simulink model "CodeGeneration"  (R2020b)
settings: Solver=FixedStepDiscrete  StartTime=0.0  StopTime=inf  FixedStep=0.001  RelTol=1e-3  EnableMultiTasking=on
undefined symbols (not defined in the file or in its folder): batch3
libraries: TIMERS_Lib x7, neural x5, USART_Lib x5, STM32_Config_Lib x2, ADC_Lib x1, simulink x1
(part 1 of 2)
settings Model: SILPILModeSetting=veronly  CodeVerificationMode=processor-in-the-loop (pil)  ExtModeTrigDuration=10  Creator=anton  LastModifiedBy=anton
settings OptimizationCC: DefaultParameterBehavior=Inlined  EnhancedBackFolding=on  PassReuseOutputArgsAs=Individual arguments  ZeroExternalMemoryAtStartup=off  ZeroInternalMemoryAtStartup=off  MaxStackSize=64  OptimizeBlockOrder=speed  DifferentSizesBufferReuse=on  OptimizationCustomize=off  EfficientTunableParamExpr=on
settings DebuggingCC: ParameterTunabilityLossMsg=error
settings HardwareCC: ProdBitPerPointer=32  ProdBitPerSizeT=32  ProdBitPerPtrDiffT=32  ProdLargestAtomicInteger=Long  ProdWordSize=32  ProdHWDeviceType=STM32CortexM
settings SFSimCC: MATLABDynamicMemAlloc=off
settings RTWCC: Description=stm32 (Embedded Target)  SystemTargetFile=stm32.tlc  TemplateMakefile=stm32.tmf  GenerateReport=on  RTWVerbose=off  Toolchain=GNU Tools for ARM Embedded Processors
settings CodeAppCC: ForceParamTrailComments=on  IgnoreCustomStorageClasses=off  MaxIdLength=64  OperatorAnnotations=on  SimulinkDataObjDesc=on  SFDataObjDesc=on  CustomSymbolStrType=$N$R$M  SimulinkBlockComments=off
settings STFCustomTargetCC: CodeReplacementLibrary=ARM CMSIS SIN COS  MultiwordLength=256  ParMdlRefBuildCompliant=on  ConcurrentExecutionCompliant=off  IncludeMdlTerminateFcn=off  CombineOutputUpdateFcns=on  ERTCustomFileBanners=on  SupportContinuousTime=off  SupportNonInlinedSFcns=off  RemoveResetFunc=on  MATLABClassNameForMDSCustomization=Simulink.SoftwareTarget.ERTCustomization  CPPClassGenCompliant=off  GRTInterface=off  SystemTargetFile=stm32.tlc
settings ERTTargetCC: CodeReplacementLibrary=ARM CMSIS SIN COS  CompOptLevelCompliant=off  ConcurrentExecutionCompliant=off  IncludeMdlTerminateFcn=off  ModelStepFunctionPrototypeControlCompliant=off  CPPClassGenCompliant=off  UseToolchainInfoCompliant=off  ExtModeStaticAllocSize=256  ExtModeMexFile=ext_serial_win32_comm  ExtModeMexArgs=0,1,115200,10  InlinedParameterPlacement=NonHierarchical  ERTSrcFileBannerTemplate=sourceFileTemplate.cgt  ERTHdrFileBannerTemplate=sourceFileTemplate.cgt  ERTDataSrcFileTemplate=sourceFileTemplate.cgt  ERTDataHdrFileTemplate=sourceFileTemplate.cgt  ERTCustomFileTemplate=customRoutineProcess.tlc

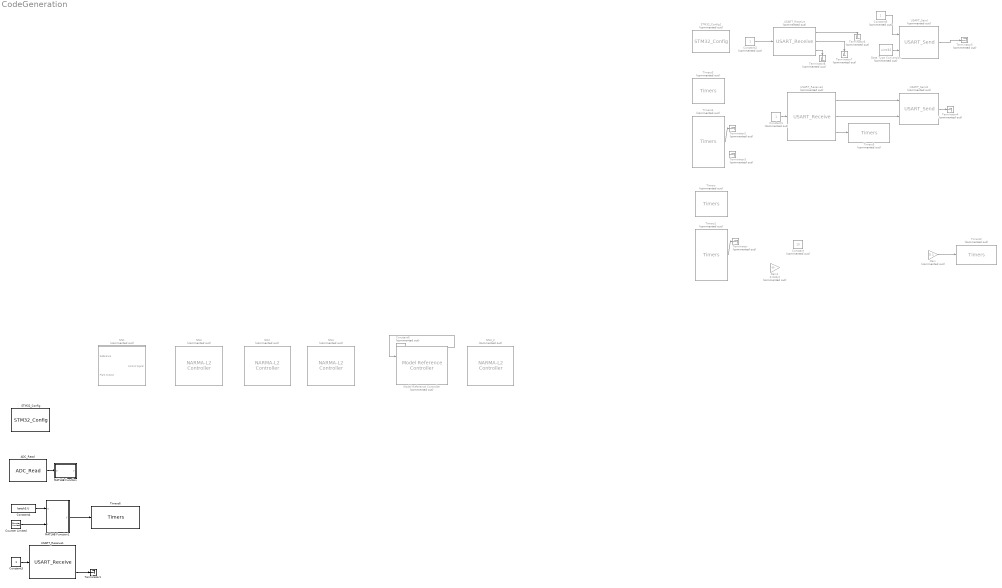
== system CodeGeneration ==
  ADC_Read : ADC_Lib/ADC_Read  ADC_Name=ADC1  ADC_Ch0=on  ADC_Ch1=off  ADC_Ch2=off  ADC_Ch3=off  ADC_Ch4=off  ADC_Ch5=off  ADC_Ch6=off  ADC_Ch7=off  ADC_Ch8=off  ADC_Ch9=off  ADC_Ch10=off  ADC_Ch11=off  ADC_Ch12=off  ADC_Ch13=off  ADC_Ch14=off  ADC_Ch15=off  ADC_Ch16=off  ADC_Ch17=off  ADC_Ch18=off  RgRk1=on  RgRk2=off  RgRk3=off  RgRk4=off  RgRk1_Ch=Ch0_r1  RgRk2_Ch=off  RgRk3_Ch=off  RgRk4_Ch=off  RgRk5=off  RgRk6=off  RgRk7=off  RgRk8=off  RgRk5_Ch=off  RgRk6_Ch=off  RgRk7_Ch=off  RgRk8_Ch=off  RgRk9=off  RgRk10=off  RgRk11=off  RgRk12=off  RgRk9_Ch=off  RgRk10_Ch=off  RgRk11_Ch=off  RgRk12_Ch=off  RgRk13=off  RgRk14=off  RgRk15=off  RgRk16=off  RgRk13_Ch=off  RgRk14_Ch=off  RgRk15_Ch=off  RgRk16_Ch=off  InjRk1=off  InjRk2=off  InjRk3=off  InjRk4=off  InjRk1_Ch=off  InjRk2_Ch=off  InjRk3_Ch=off  InjRk4_Ch=off  ADC_Trig=Not used  ADC_TrigEdge=Not used  DmaReq=off  DMA_Buffer=0  ItReq=off  AWD_Mode=NOT_USED  AWD_Ch=0  AWD_HThres=0  AWD_LThres=0  AWD_En_Int=off  AWD2_HThres=0  AWD2_LThres=0  AWD2_En_Int=off  AWD3_HThres=0  AWD3_LThres=0  AWD3_En_Int=off  EOC_SEQ=on  EOC_IT=off  JEOC_IT=off  AWD_IT=off  OVR_IT=off  CpltTrans=off  HalfTrans=off  ADC_RegNb=1  ADC_RegCh0=on  ADC_RegCh1=off  ADC_RegCh2=off  ADC_RegCh3=off  ADC_RegCh4=off  ADC_RegCh5=off  ADC_RegCh6=off  ADC_RegCh7=off  ADC_RegCh8=off  ADC_RegCh9=off  ADC_RegCh10=off  ADC_RegCh11=off  ADC_RegCh12=off  ADC_RegCh13=off  ADC_RegCh14=off  ADC_RegCh15=off  ADC_RegCh16=off  ADC_RegCh17=off  ADC_RegCh18=off  ADC_InjNb=0  ADC_InjCh0=off  ADC_InjCh1=off  ADC_InjCh2=off  ADC_InjCh3=off  ADC_InjCh4=off  ADC_InjCh5=off  ADC_InjCh6=off  ADC_InjCh7=off  ADC_InjCh8=off  ADC_InjCh9=off  ADC_InjCh10=off  ADC_InjCh11=off  ADC_InjCh12=off  ADC_InjCh13=off  ADC_InjCh14=off  ADC_InjCh15=off  ADC_InjCh16=off  ADC_InjCh17=off  ADC_InjCh18=off  NbADC=1  CurrentADC=ADC1
      settings: SourceProductName=Target Support Package - STM32 Adapter
  Constant : Constant  Commented=on  Value=10
  Constant1 : Constant  Commented=on  OutDataTypeStr=uint32
  Constant2 : Constant  Commented=on
  Constant3 : Constant  OutDataTypeStr=uint32
  Constant4 : Constant  Value=batch3.U  OutDataTypeStr=double
  Constant5 : Constant  Commented=on  OutDataTypeStr=uint32
  Constant6 : Constant  Commented=on  Value=20
  Counter Limited : simulink/Sources/Counter Limited  uplimit=15000  tsamp=0.001
  Data Type Conversion : DataTypeConversion  Commented=on  OutDataTypeStr=uint32
  Gain : Gain  Commented=on  Gain=0.1
  Gain1 : Gain  Commented=on  Gain=0.034/2
  MATLAB Function : MATLAB Function  TreatAsAtomicUnit=on  SystemSampleTime=0.001
  MATLAB Function1 : MATLAB Function  TreatAsAtomicUnit=on  SystemSampleTime=0.001
  Model Reference Controller : neural/Control Systems/Model Reference Controller  Commented=on  Nrc=[]  Nic=[]  Njc=[]  IW_y=[]  IW_u=[]  IW_r=[]  B1_c=[]  B2_c=[]  LW_c=[]  retraining_c=[]  max_i_int=0  min_i_int=0  max_r_int=[]  min_r_int=[]  Ts=0.2  S1=3  Ni=2  Nj=2  sim_file=0  trainfun=trainlm  Use_validation=1  Use_Testing=0  Use_Inc_training=[]  Use_previous_weights=1  max_i=100  min_i=0  max_r=[]  min_r=[]  sam_training=0  sam_training_c=[]  epochs=200  epochs_c=[]  minp=0  maxp=93  mint=21.399999999999998579  maxt=93  Normalize=0  IW=[-0.31575733105871184314 0.062686591686636455867;-2.3955199157333382858e-05 4.6988188726926723637e-05;0.64265348590034165888 -1.419013200965908883]  LW1_2=[-0.11494478982654444954 -0.21827174218633038638;-0.012095036588430245483 -0.011029687544739159855;1.3079273800536159733 1.1891128858228197096]  LW2_1=[-14.56571197986671784 -43.386573956542719088 0.012288416469105587631]  B1=[-7.6761807201422520563;0.70764088158851679022;0.8818915743236076521]  B2=16.065125218277426455  S1c=[]  Limit_output=0  min_output=0  max_output=0  Ref_file=0
      settings: SourceProductBaseCode=NN
  NN1 : Subsystem  Commented=on  AncestorBlock=neural/Control Systems/NARMA-L2 Controller  mask(NARMA-L2 Controller){Normalize=0, IW1_1=[0.081001796331336056722 0.15736369236145394956 -0.0061189171765253010798 0.031259373269709643528 -0.29161810270363336395 0.038960711989141236233 0.21066716241391639231 0.33564336592970134276 -0.42429187654869637836 -0.10771109383123129988 0.30271654934038322304 0.25669185229126045833 -0.18814574524270602507 -0.70360581796463639304 0.0022722054824509882454 0.22910624679545782412 0.31712007292734828434 -0.089593213208105274004 -0.29265065772660509014 0.25268525353674159417 0.40327134398474917543 0.10002475107419414591 0.10633957135057141297 0.22378520139222193852 -0.035441999466167897759 -0.09543965847989055451 -0.078475621102576539889 0.7978101624930962199 0.79197484966292575059 -0.75869567511731361709 -0.53133263705840783064 -0.40463183765462173991 1.4449740542986064806 1.423356606533091373 0.71567488745926521876 -0.71695273665588032941 -2.4976194364111630186 -0.52233538556271086328 -0.25784969469923535446 0.32001986891446365657 -0.34199391648141252986 0.21622613985873931353 0.51601933874237093658 -0.10229354784308368476 -0.063445068067935039835 0.76782685785385373922 0.58773337673444869811 -0.21322284745124506222 -1.3054574307789652554;-0.45565673055947875092 -2.8918895554005401571 -0.55732675097013917309 0.41047627061890573641 -1.0670853854999666765 -1.2269041735405823434 -0.53267398056508041826 -0.97207552132808006107 -1.5722657868604021925 -0.53941889635209872012 -0.032041342375024699229 0.09039551516666352593 -0.24629516613116916868 0.11927248975686825794 -1.2163427500639183432 0.94175325425605316276 -0.61664065600630824093 1.2537434811038190574 1.9708242434192153603 -0.18910074831646658811 1.1517160053052737378 -0.20615377037471419031 0.70037457310627138085 0.17251062422370158633 0.053382827490675487103 -1.651565422525036686 1.6906721755139886287 1.1022326413130534295 0.62515064205556036825 1.1201224089032946196 1.2824320188391788999 1.1251907270244796422 0.975294135970491749 1.2712381874161382544 1.8243027831043623355 -2.0127819149324448489 -1.9988806349665289019 0.0060280342477723233147 -0.028997473490317924455 4.2722776160136408663 0.96387017843053901522 -0.43562173505830670273 -1.0910256304234176028 -3.077903779867181111 -0.62300090522248086078 0.59335314064570743309 -0.10375978052824513798 -0.6895512783715659344 0.095697058256527731124;-0.042425975032530191533 -0.020290500259480211132 0.0020558665614247998224 -0.016851639980462271989 -9.5877759916884074858e-05 -0.00043919734009329294052 -0.02432381886257231618 -0.017583525777367700615 -0.017441386778719040335 -0.0040392297673593619001 -0.0038313554643087392899 0.0070579402620235629634 0.0078744850566811568082 -0.013939382367620677117 -0.0069330983391031903579 0.006428303090721439704 0.0076925694344603182118 -0.010213041618125990456 0.015297975743313978192 0.0069861958830649481533 -0.00039084881779854097235 -0.008621454336059724069 0.011403063240721680177 -0.027621446781558738753 0.0024782386744561469769 -0.0013077434278823262415 -0.00010498714836182009241 -0.0011898238650083332001 0.002668977180136910491 -0.00074960605879568792832 -0.0066212455474144917694 0.0036782537344367594902 0.0024779959822594154958 -0.0007716761197923681934 0.0060692515023587755713 -0.010470727481629332756 0.00651595757366603065 -0.0044179300248572807644 0.0023095130361779712264 0.0032279872975385253721 -0.0019027991455841971984 0.0030634915133303550032 -0.0039399868098482868778 -0.00029080766799168656462 0.0025879809946031118173 -0.00089996436815702825131 -0.0027431045461358116028 0.0015161575681175442926 0.00055000124936672957141;0.13973537349263717711 -0.030466654127967104926 0.13187207328935218742 0.08049426006455617788 -0.076243603851158442408 -0.16547014579527388745 -0.043008846385773881471 -0.11950007788257802077 -0.046614671001138807682 0.16047901716290213781 0.073120480998826051233 0.093856529495385407347 -0.24557469126930167591 -0.19531757450559239508 -0.25070881757410712343 -0.31477274386096759651 -0.23489476856896024382 -0.029056344281550659098 0.035279823771276613842 ...(+19340 chars)], IW3_2=[0.28221035721372655924 0.24949048164687237517 0.50091503695658035067 0.29138375416878581348 0.3047008394534790332 0.3601462353909597458 0.40525095161513946529 0.26607434365595128423 0.55636218982740370809 0.34241447621358733766 0.36922712946264368838 0.45012806085967455028 0.39746229989535664107 0.3517864672941124482 0.4414843841493564236 0.36597247241314873056 0.35722161160362497778 0.44166531166398254049 0.16265027540472642986 0.25024861114207264112 0.30989912765920363258 0.41245163179350691207 0.33932632574725996033 0.49564568667022140813 0.57942154725730332654 -0.41461285525358454462 -1.2532697594117170325 -1.016361035663570167 -0.50321252693688756086 -0.54111297537343439057 -0.64187004471658015703 -0.14877502282026722202 0.60233695514965923667 1.0051459831346829521 0.94121331461014512421 1.2528330966171683514 1.2616527525012983801 1.2522219802105709618 1.2306525532073226969 1.2285383897761898986 1.2223848740139509061 1.3599109870888566043 1.4151603107720585051 -0.24410711433607779064 -0.2618941587969862983 -0.29246174834972238354 -0.30083689664157564625 -0.3068812201344749413 -0.28850938424857819342;1.0039073009269712244 0.55909515429426293043 0.35983620274181782328 0.070909546265178188817 -0.31883710307836060638 0.021145812343666886557 -0.14052154577085901321 -0.3271388918228536058 -0.3056633047260269298 -0.1623172750176906376 0.27797165474081836356 0.15225869328795568758 0.07363456490444941771 -0.62576865843504525522 -0.049087382425018186161 -0.30920133067014099471 0.076637081473032608869 0.14304981128415980574 -0.036499429525520703244 -0.2347509035584434689 -0.26179516887628079269 0.31296574936306986725 -0.15475190365927896097 0.35308581539443995023 -0.10202609695406412993 -0.17396380085010321181 0.096710134721432985949 -0.20830070808662115578 -0.47058670424406728872 0.52295605161493230462 0.0094320573624777082067 0.06715455531127276223 0.04187265104715939823 0.30327034992914059242 0.20145747764813776159 2.0909735274704814856 0.84704439041569612456 0.50997408572182101327 0.30641972313442999987 0.19197087648156632711 -0.60791406184183405248 -0.59405380909595950634 -0.034990495138219557258 -0.069266505872329714455 0.21048086131964355294 0.22667210136932716691 0.042230258564031453172 0.03593561616959382865 0.053541505760580782036;-1.2112673056771381397 1.3552795429509238989 0.001340057277427330858 0.78347666775327995392 1.822361998970581709 0.5122989014137333541 -0.50111071047377020449 1.0617013213073929201 0.58128441457677981763 0.54344476225833260319 0.1944925038947179774 -0.43659907148292809165 1.707053424524483054 2.3777386093428747316 1.0594342712117987837 -0.35201497834900069561 -0.26906184398102572786 0.42788289669276663441 -1.4076861875310526795 0.19171855087256500783 -0.16925887294509342484 0.71966576151787531312 0.72059248245890283879 0.40053926618387347691 1.1464662234770182092 0.21463009737624402784 -0.80154327712810713447 -1.0629457174136294206 -1.0210941619912747846 -2.2004122602064311032 -1.9521985738729117354 -1.7172947022930669103 0.97621035059419447588 -0.44761702689860249915 0.77989707551171627564 0.40531267147789640237 1.1532982191938567773 1.1091066563735785255 1.4501837944712221429 1.6347891876696920566 1.3043885869211773176 1.4130197077664012895 0.91046411495307311146 -2.574445641552231212 -2.2214038450268880354 -2.6731230845813365171 -2.0029579616587414037 2.3026763340089528853 0.10442858352341162498;0.49547962694450214949 0.4634582007650282498 1.0890686566832370463 0.55177896616662225338 0.42636275537373924394 0.50771505829480712002 -0.12407657734639600255 0.32044081185938477763 0.81178540200128224136 0.43724654422399117371 -0.062071306632406897386 0.17905919149878501972 0.32630694572714147306 1.2520944876042674476 0.57891801858243330248 0.50502835376602539519 0.44893767424576869196 0.98344432483845856119 0.75591969357376931349 0.5511071553167703474 0.76629856245022498484 0.062215397882230967508 -0.15232706678745877582 -0.057308435995030514165 0.050820622281957550381 2.013762225413406437 ...(+18729 chars)], IW5_3=0.049794786120951804731, LW2_1=[0.019522040564175939525 0.010030780829141647259 -2.9269869808931687771 -0.044720248183330521541 3.3896735937268989147 0.055333660288906100222 -0.046769359291137894974 0.72657606414846986898 -0.231739559939226486 -2.8734140238129448619 -0.72738980090921023791 -3.1703753625289112783 0.030516532724820310402 -0.011164868475765466621 -2.6504898493220547806 -0.017243119800886514553 -3.6192209431664785768 0.062752740912268317741 -3.4737778709395779053 -0.020630211384971723632], LW4_3=[-0.49767595711144158033 -5.0418393908440179985 3.5744239145482166187 -3.9384524981309438907 -4.8073499402252970469 2.727310872235649164 -0.71730478292060606549 0.12740639700024902758 -4.6201956999409405924 4.0234022300950194051 5.8975918809235290396 1.9099313228049630276 0.22431709645351263771 4.1350604422295358376 3.8128713144263901569 5.2889865099553734495 5.1501748174827808313 -2.0783275816180553086 0.87022382331586878301 5.2226018567932683823], LW5_4=0.25213902069175248011, LW6_5=-0.0018683962758275409616, LW6_2=1.0196993926720294699, B1=[-13.683970472853349776;-10.829168374571350952;3.2499778850305398592;12.860073554387984274;-4.3007772967563742128;-12.715349009048415141;6.4787516301547949382;-19.564844579552055137;0.20783599937462277074;-5.7023611773114426526;10.113035508787838523;13.286447344365756251;2.8802714807787950235;26.296794390935232855;-0.69066711291984395071;-0.52575739785160779949;-8.8606049427338184898;-14.753008137324961524;1.7681866839940678648;10.252069531512537637], B2=3.7097017031416461563, B3=[0.15043469453056407259;2.9756978074974016479;7.1920582605238250196;-9.8267085343876328096;-1.1888977589751141828;-10.309826346565044375;-5.3298483838539478796;6.2524100723987032779;-3.1661464323339654214;-10.512300523957687659;-10.477978044887745313;-9.6945816023752779955;-15.116599806060138533;11.336838798593424471;11.996325424358646572;-0.47776234751081703145;6.2912996815758619462;2.9850645554334387377;2.5315214878778347085;19.896605647385079862], B4=2.3815464859015680332, Limit_output=0, min_output=0, max_output=0, Use_Previous_Weights=1, Ts=0.05, S1=20, Ni=25, Nj=25, sim_file=0, trainfun=trainlm, Use_validation=1, Use_Testing=1, max_i=100, min_i=0, max_i_int=0, min_i_int=0, sam_training=0, epochs=100, minp=4, maxp=94, mint=20.899999999999998579, maxt=94}
      mask prompts: Ts "Sample time"; trainfun "Training function"
      mask help: NARMA-L2 Controller. You first train a neural network model of the plant to be controlled. The controller is a rearrangement of the trained plant model. Double-click the NARMA-L2 Controller block to begin the plant training.
      mask init:
      | network;
      | x1 = [0    .4   NaN  .33  .55   .55  .33  .33  NaN .80  .92 .92];
      | y1 = [.95 .95 NaN  .75  .75   .55  .55  .75  NaN  .95 .95 .65];
      | x2 = [0    .43 NaN .45 .45    NaN .92 1.2 NaN .63 .85 .85 .63 .63 ];
      | y2 = [.39 .39 NaN  .41 .55   NaN .65 .65 NaN .75 .75  .55  .55  .75];
      | x3 = [.45 .45 NaN .42 .45 .48  NaN .33 .4 .33];
      | y3 = [.75 .90 NaN .83 .90 .83  NaN  .98 .95 .92];
      | x4 = [.75 .75 NaN .72 .75 .78  NaN  .5 .7 NaN .63 .7 .63];
      | y4 = [.75 .90 NaN .83 .90 .83  NaN .95 .95 NaN .98 .95 .92];
      | x5 = [.43 .43 .77 .77 .43 NaN .36 .43 .36 NaN .75 .75];
      | y5 = [.37 .41 .41 .37 .37 NaN .42 .39 .36 NaN .41 .55];
      | x6 = [.92 .92 .77 NaN .84 .77 .84];
      | y6 = [.65 .39 .39 NaN .42 .39 .36];
      | x1t=.03; y1t=.31;
      | x2t=.03; y2t=.85;
      | x8t=.03;y8t=.21;
      | x3t=.77; y3t=.53;
      | x4t=.77; y4t=.44;
      | x5t=.34; y5t=.49;
      | x6t=.58; y6t=.49;
      | 
      | 
      | t=(0:24)/24*2*pi;
      | xs = .05*cos(t);
      | ys = .05*sin(t);
      | xs1=xs+.45;
      | ys1=ys+.95;
      | xs2=xs+.75;
      | ys2=ys+.95;
      settings: OpenFcn=nncontrolutil('nnident','',gcbh,gcb,'narma_l2');
      mask Help: helpview('deeplearning','nnet_narma_l2_controller');
      mask TypeOptions trainfun: trainbfg | trainbr  | traincgb | traincgf | traincgp | traingd | traingdm | traingda | traingdx | trainlm  | trainoss | trainrp  | trainscg
      mask Display:
      | e = 0.06;
      | c1 = [120 150 230]/255;
      | c2 = ([120 150 230]+0)/383;
      | c3 = ([120 150 230]+128)/383;
      | patch([0 1 1 0],[0 0 1 1],c1);
      | patch([0 1 1 1-e 1-e 0+e],[0 0 1 1-e 0+e 0+e],c2);
      | patch([0 0 1 1-e 0+e 0+e],[0 1 1 1-e 1-e 0+e],c3);
      | plot([[x1 NaN x2]*.9-.075 ], [[y1  NaN y2]*.9-.1 ]);
      | plot([[x3 NaN xs1 NaN xs2]*.9-.075 ], [[y3 NaN ys1 NaN ys2]*.9-.1 ]);
      | plot([x4 NaN x5]*.9-.075,[y4 NaN y5]*.9-.1);
      | plot([x6 NaN ]*.9-.075,[y6 NaN ]*.9-.1);
      | plot([0 1 1 0 0],[0 0 1 1 0]);
      | text(x1t,y1t,'Plant');
      | text(x8t,y8t,'Output');
      | text(x2t,y2t,'Reference');
      | text(x3t,y3t,'Control');
      | text(x4t,y4t,'Signal');
      | text(x5t,y5t,'f');
      | text(x6t,y6t,'g');
  NN2 : neural/Control Systems/NARMA-L2 Controller  Commented=on  Normalize=0  IW1_1=[0.42999578451454106842 0.20519526356674350209 0.48560842768546641501 0.45796392885806858075 0.56450148087544238518 0.50351630398968461044 0.40693748816290253867 0.42403535086980548297 -0.58936365396049317233 -0.30903885679007220277 -0.22292526287955208297;0.25841032509566608244 -0.13737805067406735904 -0.15482151715535916181 0.65297703160385611731 0.17274411066130934689 0.40453996700577132817 -0.4111114686333410817 0.36147208605498298839 0.021131113938576966127 -0.14014771021062302769 0.092839271051875879581;-0.011434700121978670986 -0.010720729619677252242 -0.0096564374143097118919 -0.0082604891885513388045 -0.0096005768011547358565 -0.010391114612203487463 -1.0476759531353016286e-05 7.2077522336085755677e-05 -9.6420386119362220373e-05 8.2917824210678723652e-06 2.3416884195674133776e-05;-0.56744746474663465552 -0.47940353954936382186 -0.36673868830426242793 -0.72388284193056895433 -0.22890654036687180239 -0.62816667955451999106 -0.15556880492137584171 -0.27089640898497230337 -0.1535093393110727733 -0.72590483691104790154 -0.80082100631588459816;0.63814745459816246687 0.6401406546649579532 0.26654247833268734924 0.2952640512926372196 0.84955032500919014371 0.21317123129875506504 -0.29465041983107009838 -0.19037508756029189461 0.15397062431184516118 -0.07918764571200906377 -0.049066929249987248363;0.68031528203635949215 0.37921354169754795116 -0.022222469467425922524 2.0972653722608960436 0.40664857275118748703 1.4365602546419606877 0.16120398009003295003 0.033632347331193010453 -0.20163202670797347738 -0.58984661369907187556 -0.91883922634755954562]  IW3_2=[0.62072958787989240825 0.48642642668883517842 0.8143032356552284412 1.1295518407252980175 -0.12252819519746503685 1.3035863364893975902 -0.061540668235754963922 0.13396836381379054193 -0.97273489523940537271 -0.57449054628195250771 -0.79552860018882165516;0.022148742001209309471 0.35509226217601974618 0.15936552561537462025 0.41743348717457334773 0.21671159251167160242 0.21588238211386889809 0.10365014565444288785 0.32399157654972332576 -0.24370824872351357082 0.1052740296345326676 0.21533119379063728194;-0.34960873325137170609 0.60597565806765596452 1.122135647654741053 -0.20643521097916414653 0.71677006726172487472 0.30105254139888160125 -0.12032940047543728979 -0.37497085528307366742 0.34043889151749706645 -0.36823126955913926261 -0.11653268522074718139;0.19393773260013844051 0.067610881920749932306 0.23399090778869918728 0.21457707930399366747 -0.14374410046381749795 0.26692484357754975299 -0.17370341744012737784 -0.06060480970759270225 0.25309705955902561669 0.086487428730836077295 -0.042775161104023948222;0.97957315902225849946 1.1975315558082157974 0.94192073634989559316 1.2208743757048998724 1.3045447227043793781 1.0252258514225500718 0.17267256498501859507 -0.27917778045509750173 -0.21332665529313060704 -0.94663326100635658555 -1.4586763385411685157;-0.13919708229624574991 -0.04346517225565629805 -0.26370853710094882549 0.28690607977414084306 -0.38642813425088834434 -0.033589343275048713644 -0.02182821320742767135 0.0546643245090925739 -0.093743190688845248748 -0.083182309228358813913 -0.23796081789112336069]  IW5_3=0.00035625599399004379431  LW2_1=[0.0097832663468938908802 -1.6727188551373248782 4.0745823001807295327 0.70095287853249088617 -1.5696668938645457203 -0.0037480653401194630528]  LW4_3=[-1.3975705228945904945 0.5017185102204857472 2.1171483657331444661 -0.28696914872047785128 -0.97527522346300143941 0.42327247399147505114]  LW5_4=0.30108920563813407201  LW6_5=-0.64763974290970649506  LW6_2=-4.0888519730117227624  B1=[-12.820258601526894893;8.3658161662943157921;1.4697304281208545262;2.3120851336475483073;-3.5099662930913710923;-7.2883678124612831795]  B2=-2.0492682323172446424  B3=[-12.875713784252596383;-2.8354269756645469336;-6.0083619963053065405;-3.7653708851426892501;5.4665583507364479132;7.3625549242107526382]  B4=-0.58721073754749031348  Limit_output=0  min_output=0  max_output=0  Use_Previous_Weights=1  Ts=0.05  S1=6  Ni=6  Nj=6  sim_file=0  trainfun=trainlm  Use_validation=1  Use_Testing=1  max_i=100  min_i=15  max_i_int=0  min_i_int=0  sam_training=0  epochs=200  minp=18  maxp=98  mint=21.600000000000001421  maxt=98
      settings: SourceProductBaseCode=NN
  NN3 : neural/Control Systems/NARMA-L2 Controller  Commented=on  Normalize=0  IW1_1=[4.5877506179710243472 -5.8224880884168586093 -4.8116398201014956015 -1.4164815216642832052 0.81763038785532338171 -0.27198057915801182594 2.0143444159160965867 2.3407559126241523906 -1.7681452057802877764 -5.7821022484229143146 3.7430851758116423511 1.6721227367707509615 1.3289005909715654319 0.93538382702478350961 4.3919906169554563391 2.8708971599556645238 2.9337230728926533274 2.9439570630901070736 0.89485599525993375636 0.85017517791716412656 0.86891756124519170523 0.84581278816392069242 1.4448529792500321989 -2.2530121666458060581 -2.2394658222812600101 -2.2623666698858242441 -3.2386103949984401673 -2.8441633821784511049 -3.0600299960223735773;1.1720830805014157416 0.72510029776086915021 3.1152837564444717522 0.18904910378056175024 3.8224935256831891195 -1.9668126489800641377 -6.6675532679147675452 3.2650850036067073923 1.1202470114644642596 -6.2278464287587462778 3.7116215488970412117 -6.0685565334704545393 -5.0774544557597840466 -2.8632327825585677239 -0.26624337447103779697 2.8212503138002418268 -2.508547996937386948 -1.5743516070179877087 -1.3523844495695789281 -1.7764149308941030725 0.61474795424465311644 0.70076912677360470028 0.81227561839137796262 3.1740642999768993171 12.312848336435406438 12.355930113796736336 -7.2886823026066540621 -7.2809179605649720912 -7.2988342602487490396;3.0430016330075329023 2.4169740318724475259 2.4259277921412216728 4.5817733742367368066 1.8944438398997343054 1.859511580790785823 -0.53850317948302839355 -1.8306580945271937466 -1.2368319834834635706 -4.0322762699266911923 -0.2109757274893888368 1.9557147957371048275 -4.01940545609330524 -2.9868338460211498742 -2.6261247205624504986 -4.6830705275812238852 1.3397092110462973658 1.6504232012093991155 3.4069702118395546186 -3.22513040401769846 -3.4683445151905072379 -2.7658917471572559421 7.3974017903997095758 -1.5641115142871362398 3.7003543748091578536 -5.2653694153891770213 0.44047543295537849861 0.65058131350162340389 1.7225709767556538488;-4.890279222734382536 9.2820623635560259856 6.5998750720783911916 6.0323139426130865104 -5.0047680067878452803 0.4116948987745852051 -6.2914181154535384621 0.31808446778836885205 0.26438247585563112718 8.3922146620896498348 -4.7408709297709625829 2.9144904287601018922 -4.6124591317731447049 -6.1094582691993482015 -11.011217763455704244 0.27404268366330397644 0.55924390847268445892 0.46783190716662831354 0.70671702031784744413 0.73672189036226576331 0.61756628614558117807 0.78035668849300543481 0.78927769025750360576 0.81077837110447059654 0.81143931394686774627 0.74610299054055284618 0.97731444593670147025 1.0958561553222312401 0.90844578056274372102;-0.075236161728419265193 1.4529627010312577973 2.797812619081362584 3.5136868279571298324 2.7611251052148499951 2.4983963255208156973 -1.7656841404250225303 -1.9417134095882566669 -0.78088116642014793189 -1.6088640550687902664 1.7943691324232813322 0.94997145365046986587 -4.1264897357333518713 -0.026775423540358334051 -1.1477510773823724755 0.50378607124498253622 1.6560927415077055791 2.0531450920801437299 1.8745776862605858515 -2.0491210315044381396 -1.5608325026743929964 2.5284665887730941591 6.2502127026131972798 -10.694048550901566585 52.122961578317422493 53.556309256001412678 -36.106296288576920972 -36.030576479366580145 -36.593007834026053615;0.063989575652429978025 -0.041556986550670353686 -0.031083652266411285203 0.066651685652164505136 -0.041734549960076069985 -0.039025355723310617417 0.11953734079408176449 -0.085248904267280753433 -0.094181208689583476024 -0.033628899970372320982 -0.096945136753965252541 0.064131397883877019894 0.094625341370090709781 0.014827917287662261553 0.022585848901328225979 0.032759617241095002893 0.086220411041693659215 0.036976528993942395229 0.0092108912715153350853 0.06098449913498683872 0.034752769386083626202 -0.0051608948789154344278 0.0030326550159277270054 0.03485484675740441185 0.020253180352680037052 0.022824635982994119499 0.062310072838543721641 0.049798250842962854534 0.05015314426113818419 ...(+6138 chars)]  IW3_2=[0.062358389312379768066 0.059933867760648178169 0.059638039922337023058 0.039257799225629746998 -0.042892977608521710986 0.0087672609423849329202 -0.088440379294083742989 0.0043407700365922161079 -0.069881551551252293897 -0.088294496696273705449 0.041782477480814379789 0.059899181680647554937 -0.053645572449268187631 0.0028564156442049942058 0.078278081841138769104 -0.062008991991044801195 -0.053842263884374699789 -0.056195992817942741482 -0.034043222959654229065 -0.05050491174069139666 -0.038932059557208006928 -0.036324361972531811482 -0.019517496463399789525 -0.035456060620168178277 -0.012989875113196928946 -0.032487776126200282323 -0.001676689509518164943 -0.03667993303948401812 -0.029093856497292583385;0.0089341949146411227256 0.043196542765014042664 -0.046111763793666681044 -0.010471157526264679438 -0.062364231135924583227 -0.069121549529261222533 -0.060856269400886821297 -0.042418400517974581831 -0.060451262386795656667 -0.058346796047875681968 -0.079180222859112261991 0.0036802027370557398311 -0.043534445102530884564 0.0032102009835526211512 -0.017187221611705216784 0.15476161783268815864 0.12419758316213640181 0.1509952992578698916 0.14900803654666891496 0.13627369075906650697 0.11927773201766439515 0.14707599051007264057 0.13143743150228534566 0.13213462714122772845 0.13648149315145291505 0.13219979331239042897 0.1113272258290868566 0.14440329380429550721 0.142947377058244951;0.12046319339193144182 -0.052836313895128696194 -0.18981219103144658655 0.14408618432149167266 0.10276892132357731691 0.02656259847398110413 0.22292100843881473837 0.0057495277134840400146 -0.064435903389781640227 -0.0754980337842851984 -0.017866303955107208645 0.061765817288670116225 0.094341894661344016804 0.045483043120726859843 0.069462039727850921622 0.2331143029282263246 0.17268281646288186071 0.20025995022356612996 0.16257429492522024184 0.16567807576394280589 0.11476257681776874664 0.18090963329736181597 0.167073510298331257 0.14080977051149509705 0.12020884580905538686 0.14531005680825850868 0.021790618609190737232 0.11039150224340435469 0.11247882883628886053;-0.15739762904048695824 -0.25478239310084827007 -0.23853135867673710968 -0.24540693320706696845 -0.16549847789694849265 -0.27158208680699980064 -0.21228824520764491557 -0.19678463023799608322 -0.26334512571602797237 -0.26091440994101733342 -0.17703690068545505087 -0.16062972508328765553 -0.17598358115945855751 -0.1625496424016726893 -0.26635838210801798809 -0.208884459953958046 -0.1958764217202477731 -0.22208704458775718749 -0.20691536192094434066 -0.19469013205881979811 -0.18973203077934586158 -0.19296929867747744658 -0.20934125304262610201 -0.18182131675118293201 -0.57697276897127347528 -0.56119084851973710659 -0.5444357114933243702 -0.55980672953996235552 -0.54540635348844834773;0.24513278189851642197 0.20116485478010875942 0.25106234233440560821 0.16428185090259478374 0.27637620423829373228 0.30473283233506875955 0.28957088935705294075 0.31127710182372531067 0.18963656982560209152 0.28772079439633801989 0.30936472356509092663 0.27728849140228650771 0.29554353755051698815 0.25561277516872132898 0.21826262337416668657 0.2385315486962933107 0.23053664672280740899 0.23024892752520442762 0.20902791755162322684 0.23984961740448723644 0.22641550141436861399 0.23291025382129931787 0.20466253945367876566 0.16332858598416366558 0.22964847146070285766 0.23807019566036549674 0.2312341398611621468 0.20592225130579747128 0.22734686274357324143;0.10380903006185050741 -0.010075763651438730817 0.0052896867225735964835 -0.0069488036995434578069 0.073615356241652343816 0.11093664740531761215 0.1038982260322044715 0.03694189997265746872 0.047896550304743219784 0.12812174606833567903 0.13676691363433837734 0.022426014661011049039 -0.056927337711005866761 0.053972174985606441444 0.10425328952949819428 0.047670282041615913426 0.047302942221664076583 0.067193549163231794386 0.073391657383844760565 0.050650439670443012097 0.081544057044356729747 0.0792206487885007693 0.061724658743079800771 ...(+6400 chars)]  IW5_3=-0.40683118950996954855  LW2_1=[0.18367388632745329513 -0.24113376646743667209 -0.18732164710016388498 1.1048657870521041424 0.76391327859509616793 4.864930235214743881 0.59561883111477309516 -1.917303539599590323 -4.5862699562656992214 -1.1489886963737321324 0.50461435467110316022 0.48671555729633336762 0.78282586687516497737 0.17113935506526886665 -4.5042654176370335861]  LW4_3=[-0.24550482457143141257 -0.12046258227206883828 0.72278059400088856545 0.33556409988396906918 -0.20365096582041067319 -0.11065065970533820294 -0.39702006218300750495 -0.16909710388117193958 0.19457023564358214007 0.20368125579817983328 0.71902791528125675757 0.27180791243058466389 -0.62803781344313702739 1.0228245811182321567 0.24864886041124215077]  LW5_4=-0.704032194384420551  LW6_5=-0.00052115716235789574795  LW6_2=1.4812383354715947803  B1=[6.6037858506714020024;15.6190590967843832;7.2115002157788001824;4.6111630565620940203;-5.8133616172725615101;-0.61352439361774413484;-16.867912000695010732;11.523777125561503354;0.42855780624155320746;5.9314288248581084062;4.7460568926869948214;134.65286029529784173;-8.0407779755833939106;6.4517055479975411458;1.1610416736300694929]  B2=3.607603047460834933  B3=[-7.1527970321948846077;8.1273504245326648743;-6.6030087185907824221;1.1987536425192513168;-13.393850128780036002;0.62586972328921175457;1.2876737461148741737;-0.63156149919191872932;5.704177607140747952;-8.8977463766610807028;0.75364248725632110304;-11.922694834115555196;4.1889470813052707143;1.0906150890423740307;8.2092594533763563192]  B4=0.8861775603168042803  Limit_output=0  min_output=0  max_output=0  Use_Previous_Weights=1  Ts=0.05  S1=15  Ni=15  Nj=15  sim_file=0  trainfun=trainlm  Use_validation=1  Use_Testing=1  max_i=100  min_i=0  max_i_int=0  min_i_int=0  sam_training=0  epochs=200  minp=27  maxp=89  mint=20.399999999999998579  maxt=89
      settings: SourceProductBaseCode=NN
  NN3_2 : neural/Control Systems/NARMA-L2 Controller  Commented=on  Normalize=0  IW1_1=[0.039148714389914393563 0.04184575771883371903 -6.0296183153573701169e-05;-0.34244510037897918364 -0.83577023563736208001 -0.98984885365635955079]  IW3_2=[1.7482699976429136868 1.6815146793184658769 1.4643769373344286411;0.19971534547986175001 -0.23761110741996102624 -0.8313049704497363912]  IW5_3=0.0022432448317685066419  LW2_1=[2.4678568562519433982 -0.92133163820607499872]  LW4_3=[0.40163841185159132596 1.6230344928063593635]  LW5_4=-0.69253692308886294349  LW6_5=0.30756804882471866502  LW6_2=5.0314703685039310344  B1=[-2.061019820097664379;12.38881103090871072]  B2=4.1381115783143034292  B3=[11.273095141969324828;-4.8446886512396289959]  B4=0.11102912396311917509  Limit_output=0  min_output=0  max_output=0  Use_Previous_Weights=1  Ts=0.05  S1=2  Ni=2  Nj=2  sim_file=0  trainfun=trainlm  Use_validation=1  Use_Testing=1  max_i=100  min_i=0  max_i_int=0  min_i_int=0  sam_training=0  epochs=200  minp=27.030000000000001137  maxp=88.780000000000001137  mint=22.440000000000001279  maxt=88.780000000000001137
      settings: SourceProductBaseCode=NN
  NN4 : neural/Control Systems/NARMA-L2 Controller  Commented=on  Normalize=0  IW1_1=[-0.080988746250572979379 -0.13838781841168235065 -0.19464246714003791139 -0.1831737734679177998 -0.2549585151304777364 0.11295712996615900336 0.05396774551908024159 -0.084339983840538590432 -0.099785442419433004191;-0.010413890184333134126 -0.0091265575187428824022 -0.0063756329127272279994 -0.0083552108579549901057 -0.006076863504177858373 -9.7817671395440236029e-05 8.1153955099971645821e-05 9.715541730819373886e-05 1.7392127962488782369e-05;1.1513020654288714795 0.94415618342208462721 1.0375567840161767919 1.1229222945685994883 0.99225626847447712109 -0.1672127966254446374 -0.58243645017103307104 -0.43951626273631466679 -0.46180103710983733123;0.31910512731660528596 0.18870905461896675392 0.30841530355997776036 0.2982128793490136931 0.15411073386352708292 -0.029105687147781077184 -0.025462669894502486245 0.074244400452648851019 -0.17206703549074439663;0.28332045741420497365 0.25883705328865552753 0.55734588837675969053 0.45118178103568723492 1.1993033791487037742 -0.35307827846730166499 -0.046426401736290534572 -0.093962967387348550474 -0.34001905894463368973;0.63303424346071923701 0.61938341492344972661 0.67256845103291218457 0.69445647014096156813 0.75938987527353773999 0.47173708842661332685 0.485307212211659178 0.74210755204577560917 0.89534925039593660223]  IW3_2=[0.44433842822056818234 1.3308322142928747933 -0.88012309141376154908 0.10209499927550060028 -0.88668043204048252459 0.53298752161663853766 -0.016887785036579797127 -0.10699666035565690014 -0.43642222102782957105;-0.014213960576156930635 -0.98861648612602792685 0.62704188928941684278 0.19568832301796451612 0.13346564627213525212 0.1777508676739525395 0.10747435497132751259 0.34252847506430900149 -0.25680987507368963074;-0.15706502702782226821 0.18298497505928557061 0.035550919971730599034 -0.1396805708606352614 0.75028649860879381706 -0.0025150096985902493582 -0.088907366005240601181 -1.3441539181459039032 -1.3790216143720746;-0.23978469641887353858 -0.17759817661117477394 -0.17920698162589127067 -0.11455427433702475293 -0.0065057513890076018939 1.0272449657783668808 0.054508489687626650311 -0.032900514715066796201 -0.96858067035532324773;0.054410824928441445247 1.135534700071001657 -1.1676159002227570749 0.20397275271952425291 0.30242317544510588512 -0.027482815395496559829 -0.17393561909169577562 0.26424641101867157866 -0.074329744658186397421;0.08744818385947852879 0.095150012693570609756 0.059360282314576982843 -0.034850119895690243044 -0.057757247277703628596 0.2336660396468579759 0.19464318987828485574 0.15883347432507274877 -0.017678744283946268984]  IW5_3=-0.13699552970148068387  LW2_1=[1.1337981223783673013 5.2120259965505066901 0.029738112641827050414 -2.0044783267070078736 -0.034367633415846428335 -0.40681614747368238794]  LW4_3=[-2.1127949727651209599 -0.12122275336356981568 -0.91255569383502321834 0.010290064043029454807 0.66342205934284392832 0.60424499164512324167]  LW5_4=0.0076462523402957864246  LW6_5=-0.23311673795632711914  LW6_2=-4.7659452310226351202  B1=[5.5401485961125951363;1.114108857171022704;11.704355155680048028;-3.6962123711345546972;3.3365644845355144632;2.3236393221458913061]  B2=-2.2636957074711259175  B3=[-0.82079774323416199167;-1.1687681961167708522;-3.975788704779986471;4.0395617992779619954;-0.41611365491244611814;0.5011887284070680737]  B4=0.68173648090341609773  Limit_output=0  min_output=0  max_output=0  Use_Previous_Weights=1  Ts=0.2  S1=6  Ni=5  Nj=5  sim_file=0  trainfun=trainlm  Use_validation=1  Use_Testing=1  max_i=100  min_i=0  max_i_int=0  min_i_int=0  sam_training=0  epochs=100  minp=0  maxp=93  mint=21.399999999999998579  maxt=93
      settings: SourceProductBaseCode=NN
  STM32_Config : STM32_Config_Lib/STM32_Config  Priority=0  Project_Path=.\  Config_File=CodeGeneration.ioc  MCU_Name=STM32F446RETx
      settings: SourceProductName=Target Support Package - STM32 Adapter
  STM32_Config1 : STM32_Config_Lib/STM32_Config  Priority=0  Commented=on  Project_Path=.\  Config_File=CodeGeneration.ioc  MCU_Name=STM32F446RETx
      settings: SourceProductName=Target Support Package - STM32 Adapter
  Terminator{,2..8} (8 alike) : Terminator  Commented=on
  Terminator1 : Terminator
  Timers : TIMERS_Lib/Timers  Commented=on  currentTIM=none  TIM_Name=TIM1  sysUsingTimer=off  TIM_APBClock=84000000  TIM_Set_Clk=off  TIM_Prescaler=83  TIM_Clock=1000000.00  Variable_frequency=off  TIM_Set_OutFreq=off  TIM_ARR=4999  Output_frequency=200.04  Repetition_counter=0  TIM_Mode=Up  TIM_DMA=none  TIM_IRQ=off  TIM_IRQ_ONLY=off  TIM_UP=off  TIM_TRG=off  TIM_COM=off  TIM_BRK=off  NbTIM=1  CH1_enable=on  CH1N_enable=off  CH1_type=Output_PWM  CH1_DMA=off  CH1_int=off  CH1_edge=Rising  CH1_div=1  CH1_variable_duty=off  CH1_set_pulse=off  CH1_output_duty=0.20  CH1_pulse=10  CH2_enable=off  CH2N_enable=off  CH2_type=Unknown  CH2_DMA=off  CH2_int=off  CH2_edge=Rising  CH2_div=1  CH2_variable_duty=off  CH2_set_pulse=off  CH2_output_duty=0.00  CH2_pulse=0  CH3_enable=off  CH3N_enable=off  CH3_type=Unknown  CH3_DMA=off  CH3_int=off  CH3_edge=Rising  CH3_div=1  CH3_variable_duty=off  CH3_set_pulse=off  CH3_output_duty=0.00  CH3_pulse=0  CH4_enable=off  CH4N_enable=off  CH4_type=Unknown  CH4_DMA=off  CH4_int=off  CH4_edge=Rising  CH4_div=1  CH4_variable_duty=off  CH4_set_pulse=off  CH4_output_duty=0.00  CH4_pulse=0
      settings: SourceProductName=Target Support Package - STM32 Adapter
  Timers1 : TIMERS_Lib/Timers  Commented=on  currentTIM=none  TIM_Name=TIM1  sysUsingTimer=off  TIM_APBClock=84000000  TIM_Set_Clk=off  TIM_Prescaler=83  TIM_Clock=1000000.00  Variable_frequency=off  TIM_Set_OutFreq=off  TIM_ARR=1000000  Output_frequency=1.00  Repetition_counter=0  TIM_Mode=Up  TIM_DMA=none  TIM_IRQ=off  TIM_IRQ_ONLY=off  TIM_UP=off  TIM_TRG=off  TIM_COM=off  TIM_BRK=off  NbTIM=1  CH1_enable=on  CH1N_enable=off  CH1_type=Output_PWM  CH1_DMA=off  CH1_int=on  CH1_edge=Rising  CH1_div=1  CH1_variable_duty=off  CH1_set_pulse=off  CH1_output_duty=0.00  CH1_pulse=0  CH2_enable=off  CH2N_enable=off  CH2_type=Unknown  CH2_DMA=off  CH2_int=off  CH2_edge=Rising  CH2_div=1  CH2_variable_duty=off  CH2_set_pulse=off  CH2_output_duty=0.00  CH2_pulse=0  CH3_enable=off  CH3N_enable=off  CH3_type=Unknown  CH3_DMA=off  CH3_int=off  CH3_edge=Rising  CH3_div=1  CH3_variable_duty=off  CH3_set_pulse=off  CH3_output_duty=0.00  CH3_pulse=0  CH4_enable=off  CH4N_enable=off  CH4_type=Unknown  CH4_DMA=off  CH4_int=off  CH4_edge=Rising  CH4_div=1  CH4_variable_duty=off  CH4_set_pulse=off  CH4_output_duty=0.00  CH4_pulse=0
      settings: SourceProductName=Target Support Package - STM32 Adapter
  Timers2 : TIMERS_Lib/Timers  Commented=on  currentTIM=none  TIM_Name=TIM1  sysUsingTimer=off  TIM_APBClock=84000000  TIM_Set_Clk=off  TIM_Prescaler=100  TIM_Clock=831683.17  Variable_frequency=off  TIM_Set_OutFreq=off  TIM_ARR=16680  Output_frequency=49.86  Repetition_counter=0  TIM_Mode=Up  TIM_DMA=none  TIM_IRQ=off  TIM_IRQ_ONLY=off  TIM_UP=off  TIM_TRG=off  TIM_COM=off  TIM_BRK=off  NbTIM=1  CH1_enable=on  CH1N_enable=off  CH1_type=Output_PWM  CH1_DMA=off  CH1_int=off  CH1_edge=Rising  CH1_div=1  CH1_variable_duty=on  CH1_set_pulse=off  CH1_output_duty=5.00  CH1_pulse=834  CH2_enable=off  CH2N_enable=off  CH2_type=Unknown  CH2_DMA=off  CH2_int=off  CH2_edge=Rising  CH2_div=1  CH2_variable_duty=off  CH2_set_pulse=off  CH2_output_duty=0.00  CH2_pulse=0  CH3_enable=off  CH3N_enable=off  CH3_type=Unknown  CH3_DMA=off  CH3_int=off  CH3_edge=Rising  CH3_div=1  CH3_variable_duty=off  CH3_set_pulse=off  CH3_output_duty=0.00  CH3_pulse=0  CH4_enable=off  CH4N_enable=off  CH4_type=Unknown  CH4_DMA=off  CH4_int=off  CH4_edge=Rising  CH4_div=1  CH4_variable_duty=off  CH4_set_pulse=off  CH4_output_duty=0.00  CH4_pulse=0
      settings: SourceProductName=Target Support Package - STM32 Adapter
  Timers3 : TIMERS_Lib/Timers  Commented=on  currentTIM=none  TIM_Name=TIM1  sysUsingTimer=off  TIM_APBClock=84000000  TIM_Set_Clk=off  TIM_Prescaler=83  TIM_Clock=1000000.00  Variable_frequency=off  TIM_Set_OutFreq=off  TIM_ARR=4999  Output_frequency=200.04  Repetition_counter=0  TIM_Mode=Up  TIM_DMA=none  TIM_IRQ=off  TIM_IRQ_ONLY=off  TIM_UP=off  TIM_TRG=off  TIM_COM=off  TIM_BRK=off  NbTIM=1  CH1_enable=on  CH1N_enable=off  CH1_type=Output_PWM  CH1_DMA=off  CH1_int=off  CH1_edge=Rising  CH1_div=1  CH1_variable_duty=off  CH1_set_pulse=off  CH1_output_duty=0.20  CH1_pulse=10  CH2_enable=off  CH2N_enable=off  CH2_type=Unknown  CH2_DMA=off  CH2_int=off  CH2_edge=Rising  CH2_div=1  CH2_variable_duty=off  CH2_set_pulse=off  CH2_output_duty=0.00  CH2_pulse=0  CH3_enable=off  CH3N_enable=off  CH3_type=Unknown  CH3_DMA=off  CH3_int=off  CH3_edge=Rising  CH3_div=1  CH3_variable_duty=off  CH3_set_pulse=off  CH3_output_duty=0.00  CH3_pulse=0  CH4_enable=off  CH4N_enable=off  CH4_type=Unknown  CH4_DMA=off  CH4_int=off  CH4_edge=Rising  CH4_div=1  CH4_variable_duty=off  CH4_set_pulse=off  CH4_output_duty=0.00  CH4_pulse=0
      settings: SourceProductName=Target Support Package - STM32 Adapter
  Timers4 : TIMERS_Lib/Timers  Commented=on  currentTIM=none  TIM_Name=TIM1  sysUsingTimer=off  TIM_APBClock=84000000  TIM_Set_Clk=off  TIM_Prescaler=83  TIM_Clock=1000000.00  Variable_frequency=off  TIM_Set_OutFreq=off  TIM_ARR=1000000  Output_frequency=1.00  Repetition_counter=0  TIM_Mode=Up  TIM_DMA=none  TIM_IRQ=off  TIM_IRQ_ONLY=off  TIM_UP=off  TIM_TRG=off  TIM_COM=off  TIM_BRK=off  NbTIM=1  CH1_enable=on  CH1N_enable=off  CH1_type=Output_PWM  CH1_DMA=off  CH1_int=on  CH1_edge=Rising  CH1_div=1  CH1_variable_duty=off  CH1_set_pulse=off  CH1_output_duty=0.00  CH1_pulse=0  CH2_enable=off  CH2N_enable=off  CH2_type=Unknown  CH2_DMA=off  CH2_int=off  CH2_edge=Rising  CH2_div=1  CH2_variable_duty=off  CH2_set_pulse=off  CH2_output_duty=0.00  CH2_pulse=0  CH3_enable=off  CH3N_enable=off  CH3_type=Unknown  CH3_DMA=off  CH3_int=off  CH3_edge=Rising  CH3_div=1  CH3_variable_duty=off  CH3_set_pulse=off  CH3_output_duty=0.00  CH3_pulse=0  CH4_enable=off  CH4N_enable=off  CH4_type=Unknown  CH4_DMA=off  CH4_int=off  CH4_edge=Rising  CH4_div=1  CH4_variable_duty=off  CH4_set_pulse=off  CH4_output_duty=0.00  CH4_pulse=0
      settings: SourceProductName=Target Support Package - STM32 Adapter
  Timers5 : TIMERS_Lib/Timers  Commented=on  currentTIM=none  TIM_Name=TIM1  sysUsingTimer=off  TIM_APBClock=84000000  TIM_Set_Clk=off  TIM_Prescaler=100  TIM_Clock=831683.17  Variable_frequency=off  TIM_Set_OutFreq=off  TIM_ARR=16680  Output_frequency=49.86  Repetition_counter=0  TIM_Mode=Up  TIM_DMA=none  TIM_IRQ=off  TIM_IRQ_ONLY=off  TIM_UP=off  TIM_TRG=off  TIM_COM=off  TIM_BRK=off  NbTIM=1  CH1_enable=on  CH1N_enable=off  CH1_type=Output_PWM  CH1_DMA=off  CH1_int=off  CH1_edge=Rising  CH1_div=1  CH1_variable_duty=on  CH1_set_pulse=off  CH1_output_duty=5.00  CH1_pulse=834  CH2_enable=off  CH2N_enable=off  CH2_type=Unknown  CH2_DMA=off  CH2_int=off  CH2_edge=Rising  CH2_div=1  CH2_variable_duty=off  CH2_set_pulse=off  CH2_output_duty=0.00  CH2_pulse=0  CH3_enable=off  CH3N_enable=off  CH3_type=Unknown  CH3_DMA=off  CH3_int=off  CH3_edge=Rising  CH3_div=1  CH3_variable_duty=off  CH3_set_pulse=off  CH3_output_duty=0.00  CH3_pulse=0  CH4_enable=off  CH4N_enable=off  CH4_type=Unknown  CH4_DMA=off  CH4_int=off  CH4_edge=Rising  CH4_div=1  CH4_variable_duty=off  CH4_set_pulse=off  CH4_output_duty=0.00  CH4_pulse=0
      settings: SourceProductName=Target Support Package - STM32 Adapter
  Timers6 : TIMERS_Lib/Timers  currentTIM=TIM1  TIM_Name=TIM1  sysUsingTimer=off  TIM_APBClock=84000000  TIM_Set_Clk=off  TIM_Prescaler=1  TIM_Clock=42000000.00  Variable_frequency=off  TIM_Set_OutFreq=off  TIM_ARR=10000  Output_frequency=4200.00  Repetition_counter=0  TIM_Mode=Up  TIM_DMA=none  TIM_IRQ=off  TIM_IRQ_ONLY=off  TIM_UP=off  TIM_TRG=off  TIM_COM=off  TIM_BRK=off  NbTIM=1  CH1_enable=on  CH1N_enable=off  CH1_type=Output_PWM  CH1_DMA=off  CH1_int=off  CH1_edge=Rising  CH1_div=1  CH1_variable_duty=on  CH1_set_pulse=off  CH1_output_duty=0.00  CH1_pulse=0  CH2_enable=off  CH2N_enable=off  CH2_type=Unknown  CH2_DMA=off  CH2_int=off  CH2_edge=Rising  CH2_div=1  CH2_variable_duty=off  CH2_set_pulse=off  CH2_output_duty=0.00  CH2_pulse=0  CH3_enable=off  CH3N_enable=off  CH3_type=Unknown  CH3_DMA=off  CH3_int=off  CH3_edge=Rising  CH3_div=1  CH3_variable_duty=off  CH3_set_pulse=off  CH3_output_duty=0.00  CH3_pulse=0  CH4_enable=off  CH4N_enable=off  CH4_type=Unknown  CH4_DMA=off  CH4_int=off  CH4_edge=Rising  CH4_div=1  CH4_variable_duty=off  CH4_set_pulse=off  CH4_output_duty=0.00  CH4_pulse=0
      settings: SourceProductName=Target Support Package - STM32 Adapter
  USART_Receive : USART_Lib/USART_Receive  Commented=on  USART_name=USART2  Buff_size=512  nbUsart=1  Soft_it=off  Soft_num=0  usartMode=Asynchronous  usartDma_Rx=off  usartDma_Tx=off  usartIt=off
      settings: SourceProductName=Target Support Package - STM32 Adapter
  USART_Receive1 : USART_Lib/USART_Receive  USART_name=USART2  Buff_size=1  nbUsart=1  Soft_it=on  Soft_num=0  usartMode=Asynchronous  usartDma_Rx=off  usartDma_Tx=off  usartIt=off
      settings: SourceProductName=Target Support Package - STM32 Adapter
  USART_Receive2 : USART_Lib/USART_Receive  Commented=on  USART_name=USART2  Buff_size=1  nbUsart=1  Soft_it=on  Soft_num=0  usartMode=Asynchronous  usartDma_Rx=off  usartDma_Tx=off  usartIt=off
      settings: SourceProductName=Target Support Package - STM32 Adapter
  USART_Send : USART_Lib/USART_Send  Commented=on  USART_name=USART2  Buff_size=32  nbUsart=1  usartMode=Asynchronous  usartDma_Rx=off  usartDma_Tx=off  usartIt=off
      settings: SourceProductName=Target Support Package - STM32 Adapter
  USART_Send1 : USART_Lib/USART_Send  Commented=on  USART_name=USART2  Buff_size=32  nbUsart=1  usartMode=Asynchronous  usartDma_Rx=off  usartDma_Tx=off  usartIt=off
      settings: SourceProductName=Target Support Package - STM32 Adapter
  wires:
  Constant3/1 -> USART_Receive1/1
  USART_Send/1 -> Terminator5/1
  Timers1/1 -> Terminator/1
  ? -> Gain1/1
  USART_Receive2/2 -> USART_Send1/2
  USART_Receive2/1 -> USART_Send1/1
  Timers4/1 -> Terminator2/1
  Constant1/1 -> USART_Receive2/1
  ? -> Terminator3/1
  USART_Send1/1 -> Terminator4/1
  USART_Receive2/3 -> Timers5/1
  Gain/1 -> Timers2/1
  USART_Receive1/3 -> Terminator1/1
  ADC_Read/1 -> MATLAB Function/1(u)
  USART_Receive/3 -> Terminator8/1
  Constant4/1 -> MATLAB Function1/1(u)
  USART_Receive/1 -> Terminator6/1
  Counter Limited/1 -> MATLAB Function1/2(i)
  USART_Receive/2 -> Terminator7/1
  Constant2/1 -> USART_Receive/1
  Constant5/1 -> USART_Send/1
  Data Type Conversion/1 -> USART_Send/2
  Constant6/1 -> Model Reference Controller/1
  MATLAB Function1/1(y) -> Timers6/1
